simulink library "libreria_comunicaciones_cliente2"  (R2018a)
settings: Solver=VariableStepAuto  StartTime=0.0  StopTime=10.0  RelTol=1e-3
undefined symbols (not defined in the file or in its folder): Ts
libraries: simulink x1
settings Model: Creator=ana-n  LastModifiedBy=ana-n
settings CodeAppCC: StateflowObjectComments=on

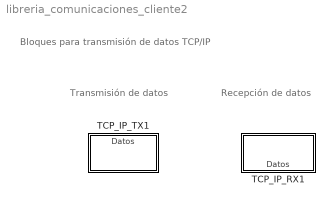
== system libreria_comunicaciones_cliente2 ==
  note: Bloques para transmisión de datos TCP/IP
  note: Recepción de datos
  note: Transmisión de datos
  TCP_IP_RX1 : Subsystem
      mask Display: disp('TCP_IP_RX')
  TCP_IP_TX1 : Subsystem
      mask Display: disp('TCP_IP_TX');

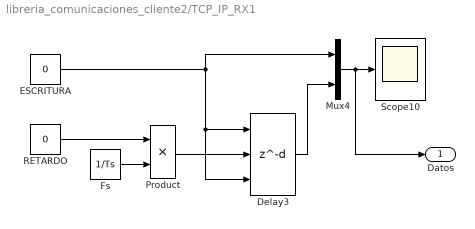
== system libreria_comunicaciones_cliente2/TCP_IP_RX1 ==
  Delay3 : Delay  DelayLengthSource=Input port  DelayLength=1  DelayLengthUpperLimit=1000  InitialConditionSource=Input port  InitialCondition=0  InputProcessing=Inherited
      settings: InputPortMap=u0,p1,p4
  ESCRITURA : Constant  Value=0
  Fs : Constant  Value=1/Ts
  Mux4 : Mux  Inputs=2
  Product : Product
  RETARDO : Constant  Value=0
  Scope10 : Scope
  Datos : Outport
  wires:
  Product/1 -> Delay3/2
  Delay3/1 -> Mux4/2
  RETARDO/1 -> Product/1
  Fs/1 -> Product/2
  ESCRITURA/1 -> Delay3/3, Delay3/1, Mux4/1
  Mux4/1 -> Datos/1, Scope10/1

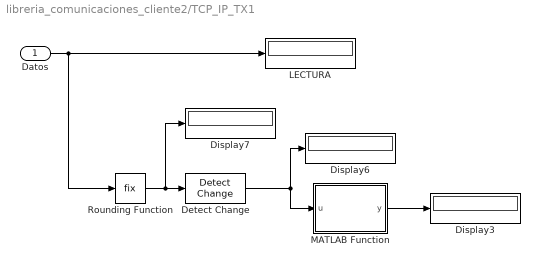
== system libreria_comunicaciones_cliente2/TCP_IP_TX1 ==
  Datos : Inport
  Detect Change : simulink/Logic and Bit Operations/Detect Change  vinit=0  OutDataTypeStr=boolean
  Display3 : Display
  Display6 : Display
  Display7 : Display
  LECTURA : Display
  MATLAB Function : MATLAB Function  TreatAsAtomicUnit=on
  Rounding Function : Rounding  Operator=fix
  wires:
  Rounding Function/1 -> Display7/1, Detect Change/1
  MATLAB Function/1(y) -> Display3/1
  Detect Change/1 -> MATLAB Function/1(u), Display6/1
  Datos/1 -> Rounding Function/1, LECTURA/1

== matlab function libreria_comunicaciones_cliente2/TCP_IP_TX1/MATLAB Function ==
  data: u input; y output
%Esta función envía y recibos los datos
%desde el CCL a través del script_ciclo_vs.m
function y = fcn(u)
    coder.extrinsic('run')
    if u==1
        run script_ciclo_vs2.m
        y=1;
    else
        y=0;
    end
end
